simulink model "samolot"  (R2025a)
settings: Solver=VariableStepAuto  StartTime=0.0  StopTime=10.0  RelTol=1e-3
values from neighbouring files (symbols this model uses):
  h = 42    [zad1.m]
  k1 = 54.7    [zad1.m]
  k2 = 303.6    [zad1.m]
  m1 = 14000    [zad1.m]
  m2 = 450.28    [zad1.m]
  m3 = 200    [zad1.m]
settings Model: Creator=D106-Student  LastModifiedBy=Dejmian

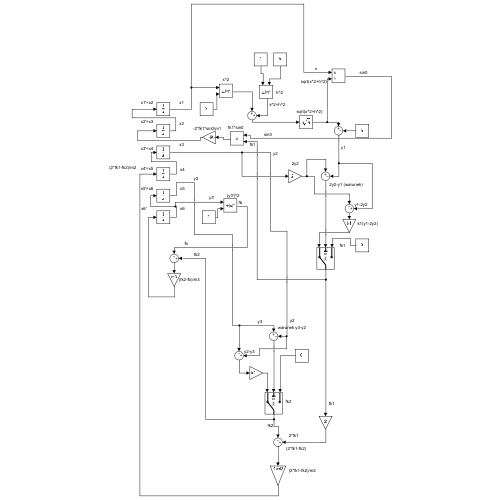
[thumbnail: Simulink's stored preview of the top-level diagram]
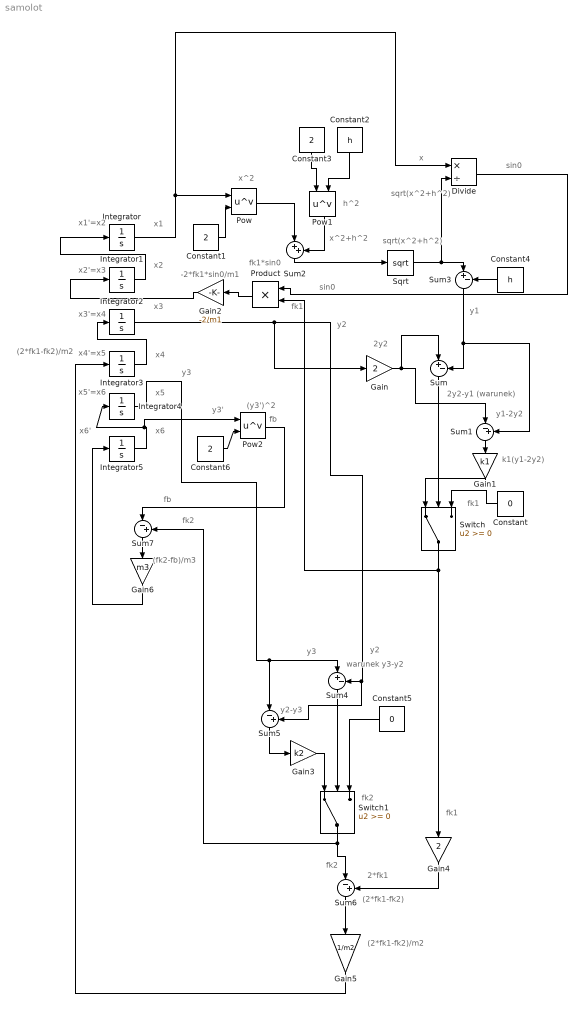
== system samolot ==
  note: (fk2-fb)/m3
  note: fk2
  note: fb
  note: fb
  note: (y3')^2
  note: (2*fk1-fk2)/m2
  note: (2*fk1-fk2)
  note: fk2
  note: 2*fk1
  note: fk1
  note: y2-y3
  note: fk2
  note: y2
  note: y3
  note: warunek y3-y2
  note: sin0
  note: fk1
  note: sqrt(x^2+h^2)
  note: x
  note: -2*fk1*sin0/m1
  note: fk1*sin0
  note: sin0
  note: fk1
  note: k1(y1-2y2)
  note: y1-2y2
  note: 2y2-y1 (warunek)
  note: 2y2
  note: y1
  note: sqrt(x^2+h^2)
  note: x^2+h^2
  note: h^2
  note: x^2
  note: y3'
  note: y3
  note: y2
  note: x6'
  note: x6
  note: x5'=x6
  note: x5
  note: x4'=x5
  note: x4
  note: x3'=x4
  note: x3
  note: x2'=x3
  note: x2
  note: x1'=x2
  note: x1
  note: (2*fk1-fk2)/m2
  Constant : Constant  Value=0
  Constant1 : Constant  Value=2
  Constant2 : Constant  Value=h
  Constant3 : Constant  Value=2
  Constant4 : Constant  Value=h
  Constant5 : Constant  Value=0
  Constant6 : Constant  Value=2
  Divide : Product  Inputs=*/
  Gain : Gain  Gain=2
  Gain1 : Gain  Gain=k1
  Gain2 : Gain  Gain=-2/m1
  Gain3 : Gain  Gain=k2
  Gain4 : Gain  Gain=2
  Gain5 : Gain  Gain=1/m2
  Gain6 : Gain  Gain=m3
  Integrator{,2..5} (5 alike) : Integrator
  Integrator1 : Integrator  InitialCondition=67
  Pow : Math  Operator=pow  SignedPower=on  RndMeth=Zero
  Pow1 : Math  Operator=pow  SignedPower=on  RndMeth=Zero
  Pow2 : Math  Operator=pow  SignedPower=on  RndMeth=Zero
  Product : Product
  Sqrt : Sqrt
  Sum : Sum  Inputs=|+-
  Sum{1,5..7} (4 alike) : Sum  Inputs=|-+
  Sum2 : Sum  Inputs=|++
  Sum3 : Sum  Inputs=|+-
  Sum4 : Sum  Inputs=|+-
  Switch : Switch  SaturateOnIntegerOverflow=off  InputSameDT=off
  Switch1 : Switch  SaturateOnIntegerOverflow=off  InputSameDT=off
  wires:
  Integrator5/1 -> Pow2/1, Integrator4/1
  Integrator3/1 -> Integrator2/1
  Integrator4/1 -> Sum5/1, Sum4/1
  Pow/1 -> Sum2/1
  Pow1/1 -> Sum2/2
  Sum2/1 -> Sqrt/1
  Constant4/1 -> Sum3/2
  Sqrt/1 -> Divide/2, Sum3/1
  Sum3/1 -> Sum1/2, Sum/2
  Gain/1 -> Sum1/1, Sum/1
  Sum1/1 -> Gain1/1
  Integrator/1 -> Pow/1, Divide/1
  Divide/1 -> Product/1
  Switch/1 -> Gain4/1, Product/2
  Product/1 -> Gain2/1
  Gain2/1 -> Integrator1/1
  Integrator2/1 -> Sum5/2, Sum4/2, Gain/1
  Constant3/1 -> Pow1/1
  Constant2/1 -> Pow1/2
  Constant1/1 -> Pow/2
  Sum/1 -> Switch/2
  Gain1/1 -> Switch/1
  Constant/1 -> Switch/3
  Sum4/1 -> Switch1/2
  Constant5/1 -> Switch1/3
  Sum5/1 -> Gain3/1
  Gain3/1 -> Switch1/1
  Switch1/1 -> Sum6/1, Sum7/2
  Gain4/1 -> Sum6/2
  Sum6/1 -> Gain5/1
  Gain5/1 -> Integrator3/1
  Constant6/1 -> Pow2/2
  Pow2/1 -> Sum7/1
  Sum7/1 -> Gain6/1
  Gain6/1 -> Integrator5/1
  Integrator1/1 -> Integrator/1
